simulink model "simulator_prototype"  (R2021b)
(part 12 of 12)

et761 = (t2307.*(-t6196+t6428+t3055.*(-t4494-t4495+t4799+t4823+t3976.*(t2694-t2701+t3036-t3043).*4.0e-8+t3980.*(t2694-t2701+t3036-t3043).*2.4e-7)))./2.0+(t7799.*(t1861-t3221))./2.0+(t3216.*(-t5828-t5829+t6593+t6596+t22.*t6699.*(t3242-t3554)+t28.*t6696.*(t3242-t3554)))./2.0;
et762 = (t3503.*(t6287+t4031.*(t4795+t4801+t4808+t3976.*(t2694-t2701+t3036-t3043).*5.7e-7)+t4026.*(-t4494-t4495+t4799+t4823+t3976.*(t2694-t2701+t3036-t3043).*4.0e-8+t3980.*(t2694-t2701+t3036-t3043).*2.4e-7)))./2.0;
et763 = (t3915.*(t6872+t6058.*(t1896-t3239)+t4019.*(t3435-t3448+t4615+t4619+t3976.*(t1896-t3239).*5.7e-7+t3980.*(t1896-t3239).*4.0e-8)))./2.0;
et764 = (t3217.*(t6251-t6997-t7310+t7388+t7554+t4880.*(t3435-t3448+t4615+t4619+t3976.*(t1896-t3239).*5.7e-7+t3980.*(t1896-t3239).*4.0e-8)))./2.0+t4215.*t5279.*(t2694-t2701+t3036-t3043).*5.43845e-3;
et765 = t3810.*t6011.*(t2694-t2701+t3036-t3043).*5.43845e-3+t3951.*t6647.*(t2694-t2701+t3036-t3043).*3.633675e-3+t3810.*t3934.*(et753+et754+et755+et756).*5.43845e-3+et757.*et758+t3934.*t5771.*(t1513+t1879+t2598+t2820+t2834+t3117+t3118).*3.633675e-3;
et766 = t50.*t189.*(t5618+t6429-t6902+t3055.*(t4795+t4801+t4808+t3976.*(t2694-t2701+t3036-t3043).*5.7e-7)+t6384.*(t1477-t2502)).*4.771516396025243e-17;
et767 = t5309+t5438+t6275+t6278+t7019+t7027+t7575+t7577-t7579+t7723+t7781+t7783+t7811-t7813-t7907+t7934-t7936+(t2994.*(-t6772+t6776+t3055.*(-t3434+t4606+t3980.*(t1896-t3239).*1.02e-6)))./2.0+(t7461.*(t1456-t2355))./2.0+(t7524.*(t11.*((t237.*(t42-t43))./9.007199254740992e+15+t15.*(-t1881+t3121+t3276))+t16.*(-t1901+t3122+t3277)))./2.0;
et768 = (t3047.*(t6462-t6464-t6766-t6767+t3055.*(t4809+t3976.*(t2694-t2701+t3036-t3043).*1.02e-6)+t5572.*(t1477-t2502)))./2.0;
et769 = t3704+t3707-t3863+t4904+t4912-t5154+t5155-t5186+t3370.*(t1477-t2502).*9.3e-7+t4031.*(t3512-t4006).*9.0e-8+t12.*t3980.*(t3242-t3554).*9.0e-8;
et770 = t17.*t3980.*(t3242-t3554).*9.3e-7;
et771 = t6736+t6778+t6779+t6783+t6787-t7024-t7025+t7205+t7207+t7398+(t3395.*(et769+et770))./2.0+(t5857.*(t4673+t2363.*(t3566.*1.838876e-2+t4109-t4110+t28.*(t1896-t3239).*9.99471e-3).*7.26735e-3))./2.0+(t5792.*(t1477-t2502))./2.0;
et772 = (t3055.*(t4876+t4905+t4906+t3055.*(t1456-t2355).*1.02e-6+t3047.*(t1477-t2502).*1.02e-6+t3976.*(t3242-t3554).*1.02e-6))./2.0;
et773 = t3704+t3707-t3863+t4904+t4912-t5154+t5155-t5186+t3370.*(t1477-t2502).*9.3e-7+t4031.*(t3512-t4006).*9.0e-8+t12.*t3980.*(t3242-t3554).*9.0e-8;
et774 = t17.*t3980.*(t3242-t3554).*9.3e-7;
et775 = t6738+t6778+t6779+t6783+t6787-t7024-t7025+t7205+t7207+t7398+(t3395.*(et773+et774))./2.0+(t5858.*(t4673+t2363.*(t3566.*1.838876e-2+t4109-t4110+t28.*(t1896-t3239).*9.99471e-3).*7.26735e-3))./2.0+(t5792.*(t1477-t2502))./2.0;
et776 = (t3055.*(t4876+t4905+t4906+t3055.*(t1456-t2355).*1.02e-6+t3047.*(t1477-t2502).*1.02e-6+t3976.*(t3242-t3554).*1.02e-6))./2.0;
et777 = t707+t708-t721-t722-t749+t762+t768-t777-t792-t793-t801-t802-t808+t813-t819+t821-t1629+t1637-t1640-t1641-t1659-t1661+t1666+t1667+t1683+t1692+t1705-t1712+t1758+t1759+t1775+t1776+t1973+t1993+t1994+t2023+t2053+t2060-t2089-t2090+t2098+t2099-t8.*t9.*t15.*t50.*t189.*3.670836568391568e-22;
et778 = t10.*t13.*t14.*t50.*t189.*(-3.279367663374749e-19)-t8.*t9.*t11.*t15.*t50.*t189.*7.075931802640439e-19;
et779 = t8.*t11.*t14.*t15.*t50.*t189.*(-1.190170786299927e-18)-t9.*t11.*t13.*t15.*t50.*t189.*1.190170786299927e-18;
et780 = t13.*t14.*t15.*t16.*t50.*t189.*(-3.226512155691387e-19);
et781 = -t5343-t5565-t5813-t5851+t5876-t5880+t6066+t6095+t6174+t6223-t6425+t6460-t6469+t6482+t6702+t6708-t6962-t6964+t6995+t7114-t7159-t7161+t7420;
et782 = (t5278.*(t350+t366-t1205+t1210-t1217-t1218-t2147+t2152+t2154+t2155-t3405-t3409-t3420-t3739+t3746+t26.*t50.*t202.*(t46-t47).*8.687615694748404e-39))./2.0;
et783 = (t3500.*(t4573.*(t2813-t2835+t12.*(t1456-t2355).*1.02e-6+t17.*(t1456-t2355).*9.0e-8)+t4577.*(-t2804+t2838+t3109+t17.*(t1456-t2355).*9.3e-7)+t3133.*(t3242-t3554)))./2.0+(t5026.*(et777+et778+et779+et780))./2.0+(t6916.*(t1861-t3221))./2.0;
et784 = (t6647.*(t3359-t3670+t22.*(t3242-t3554).*1.33637554986e-4+t28.*(t3242-t3554).*7.26350557185e-5))./2.0+(t3502.*(t3993+t4240-t4332+t4464+t4031.*(t2801-t2850)+t4026.*(t335-t1539-t2831+t2851)))./2.0;
et785 = (t5949.*(t4843+t5108+t2307.*(t642+t643-t667+t674+t1587+t1606+t1608+t1609+t2295+t2671+t2683+t2684-t2695+t3279+t3297-t3303+t3597+t3603+t3609-t3614+t4053+t4054)+t2297.*(t2292+t3290+t3524.*1.838876e-2-t3591+t3592+t3611+t16.*(t1861-t3221).*3.131399999999998e-4+t16.*t17.*(t1861-t3221).*9.99471e-3)))./2.0;
et786 = t1288+t1289+t1302+t1303-t1319-t1320+t1336-t1348+t1350+t1351-t1360+t1369-t1378+t1396-t1425+t1435-t2174+t2183-t2187+t2193-t2194-t2195+t2199-t2203-t2215+t2219-t2222-t2223+t2239+t2240-t2256-t2257+t2555+t2556+t2572+t2583-t2605-t2606+t2612+t2613-t2618-t2619+t2651+t2652;
et787 = t18.*t19.*t20.*t50.*t202.*(-3.566935413776081e-21);
et788 = t24.*t25.*t26.*t50.*t202.*(-3.992732227073824e-24);
et789 = t18.*t19.*t26.*t27.*t50.*t202.*(-3.509445006623964e-21);
et790 = t21.*t24.*t25.*t26.*t50.*t202.*(-7.696420262413979e-21);
et791 = -t5430+t5493-t5496+t6086-t6112+t6149+t6151./2.0+t6156-t6192+t6194-t6231+t6237+t6283+t6580+t6594+t6611+t6613-t6645-t6648-t6705-t6742+t6744-t7118-t7125+t7170+t7176-t7326+t7328+t7410+(t4950.*(et786+et787+et788+et789+et790))./2.0+(t7092.*(t1477-t2502))./2.0;
et792 = (t3055.*(t3131+t3132+t3171+t3446-t4281-t4282-t4301+t4303-t4308+t4310-t4583-t4594+t4623+t4639+t2388.*(t1456-t2355).*4.0e-8+(t3543.*(t1861-t3221))./1.0e+8+(t3500.*(t1896-t3239))./1.0e+8-t11.*t2297.*t2363.*2.4e-7))./2.0;
et793 = (t2363.*(t3157+t3158+t3386-t4299-t4300-t4562+t4567+t3543.*(t1861-t3221).*6.2e-7+t3500.*(t1896-t3239).*6.2e-7-(t11.*(t1861-t3221).*(t1896-t3239))./1.0e+8-(t11.*t2297.*t2363)./1.0e+8-(t11.*t3502.*t3547)./1.0e+8))./2.0+(t5859.*(t4927+t5198-t5762-t6392))./2.0;
et794 = (t21.*t2363.*(-t3434+t4606+t3980.*(t1896-t3239).*1.02e-6))./2.0;
et795 = t1288+t1289+t1302+t1303-t1319-t1320+t1336-t1348+t1350+t1351-t1360+t1369-t1378+t1396-t1425+t1435-t2174+t2183-t2187+t2193-t2194-t2195+t2199-t2203-t2215+t2219-t2222-t2223+t2239+t2240-t2256-t2257+t2555+t2556+t2572+t2583-t2605-t2606+t2612+t2613-t2618-t2619+t2651+t2652;
et796 = t18.*t19.*t20.*t50.*t202.*(-3.566935413776081e-21);
et797 = t24.*t25.*t26.*t50.*t202.*(-3.992732227073824e-24);
et798 = t18.*t19.*t26.*t27.*t50.*t202.*(-3.509445006623964e-21);
et799 = t21.*t24.*t25.*t26.*t50.*t202.*(-7.696420262413979e-21);
et800 = -t5430+t5493-t5496+t6086-t6112+t6149+t6151./2.0+t6156-t6192+t6194-t6233+t6239+t6283+t6580+t6594+t6611+t6613-t6646-t6649-t6705-t6742+t6744-t7118-t7125+t7170+t7176-t7326+t7328+t7412+(t4950.*(et795+et796+et797+et798+et799))./2.0+(t7092.*(t1477-t2502))./2.0;
et801 = (t3055.*(t3131+t3132+t3171+t3446-t4281-t4282-t4301+t4303-t4308+t4310-t4583-t4594+t4623+t4639+t2388.*(t1456-t2355).*4.0e-8+(t3543.*(t1861-t3221))./1.0e+8+(t3500.*(t1896-t3239))./1.0e+8-t11.*t2297.*t2363.*2.4e-7))./2.0;
et802 = (t2363.*(t3157+t3158+t3386-t4299-t4300-t4562+t4567+t3543.*(t1861-t3221).*6.2e-7+t3500.*(t1896-t3239).*6.2e-7-(t11.*(t1861-t3221).*(t1896-t3239))./1.0e+8-(t11.*t2297.*t2363)./1.0e+8-(t11.*t3502.*t3547)./1.0e+8))./2.0+(t5860.*(t4927+t5198-t5762-t6392))./2.0;
et803 = (t21.*t2363.*(-t3434+t4606+t3980.*(t1896-t3239).*1.02e-6))./2.0;
et804 = -t5344-t5568+t5679+t5689+t5925+t5927-t5966+t5976+t5980-t6241+t6295+t6367+t6528+t6540+t7028+t7031-t7040+t7300+t7302-t7363+t7612+t7616;
et805 = (t4118.*(t4573.*(t2813-t2835+t12.*(t1456-t2355).*1.02e-6+t17.*(t1456-t2355).*9.0e-8)+t4577.*(-t2804+t2838+t3109+t17.*(t1456-t2355).*9.3e-7)+t3133.*(t3242-t3554)))./2.0;
et806 = (t6651.*(t4814.*(t1861-t3221)+t2297.*(t642+t643-t667+t674+t1587+t1606+t1608+t1609+t2295+t2671+t2683+t2684-t2695+t3279+t3297-t3303+t3597+t3603+t3609-t3614+t4053+t4054)))./2.0+(t5809.*(t951+t10.*(-t1881+t3121+t3276)))./2.0+((t1861-t3221).*(t4658+t4719+t5240+t5262-t3483.*(t1005+t20.*(t1941-t3315+t39.*t1022.*(t855-t878).*2.196325630278387e-1))-t3431.*(t1896-t3239)))./2.0+(t3808.*t5645.*(t2674-t2676+t3022-t3027))./2.0;
et807 = (t3925.*t5946.*(t2674-t2676+t3022-t3027))./2.0;
et808 = -t5344-t5568+t5679+t5689+t5925+t5927-t5966+t5978+t5980-t6241+t6299+t6367+t6528+t6540+t7028+t7031-t7040+t7300+t7302-t7363+t7614+t7618;
et809 = (t4118.*(t4573.*(t2813-t2835+t12.*(t1456-t2355).*1.02e-6+t17.*(t1456-t2355).*9.0e-8)+t4577.*(-t2804+t2838+t3109+t17.*(t1456-t2355).*9.3e-7)+t3133.*(t3242-t3554)))./2.0;
et810 = (t6651.*(t4814.*(t1861-t3221)+t2297.*(t642+t643-t667+t674+t1587+t1606+t1608+t1609+t2295+t2671+t2683+t2684-t2695+t3279+t3297-t3303+t3597+t3603+t3609-t3614+t4053+t4054)))./2.0+(t5809.*(t951+t10.*(-t1881+t3121+t3276)))./2.0+((t1861-t3221).*(t4658+t4719+t5240+t5262-t3483.*(t1005+t20.*(t1941-t3315+t39.*t1022.*(t855-t878).*2.196325630278387e-1))-t3431.*(t1896-t3239)))./2.0+(t3808.*t5646.*(t2674-t2676+t3022-t3027))./2.0;
et811 = (t3925.*t5949.*(t2674-t2676+t3022-t3027))./2.0;
et812 = t5456+t5457+t7237+t7242+t7246+t7250+t7453+t7498+t7502+t7546+t7701+t7740+t7741-t7766+t7833+(t3047.*(t5490+t6190-t6193-t6609-t6610+t5405.*(t1477-t2502)))./2.0+(t3991.*(t5713+t5714-t6443-t6719-t6722+t6102.*(t3563-t4051)))./2.0+(t3980.*(t5691+t6884-t6886-t7353-t7354+t6065.*(t3242-t3554)))./2.0+(t7426.*(t1456-t2355))./2.0+(t3991.*(t6263-t6887+t6888-t7355+t7307.*(t3563-t4051)+t21.*t3547.*(-t3434+t4606+t3980.*(t1896-t3239).*1.02e-6)))./2.0;
et813 = (t11.*t7523.*(t1861-t3221))./2.0;
et814 = t31.*(et710+et711+et712+et713+et714+et715+et716+et717+et718+et719+et720+et721+et722+et723+et724+et725)+t29.*t7835+t30.*t7836+t32.*(et730+et731+et732+et733+et734+et735+et736+et737+et738+et739)-t33.*(et747+et748+et749+et750);
et815 = -t34.*(t7589+t7647+t7648+t7861+t7891+t7892-(t2297.*t7796)./2.0+(t3047.*t7714)./2.0-(t3502.*t7826)./2.0-(t3980.*t7755)./2.0-(t3991.*t7756)./2.0+((t1861-t3221).*(t7182-t7187+t4577.*(t3846-t5169-t5184+t5185+t3055.*(t2337+t12.*(t1456-t2355)).*9.3e-7+t4553.*(t3242-t3554).*9.3e-7)+t4573.*(t3840+t3862-t5164+t5167-t5183+t5189)))./2.0)+dq3.*dq4.*(et759+et760+et761+et762+et763+et764+et765+et766);
et816 = -dq3.*dq6.*(et767+et768)-dq1.*dq6.*(et771+et772)-dq2.*dq6.*(et775+et776)-dq5.*dq6.*(t5370-t5372-t7256+t7260+t7264+t7719+t7771+(t7755.*(t1861-t3221))./2.0+(t6711.*(t4675-t5454))./2.0).*2.0+dq3.*dq4.*(t4559+t4713+t5283+t5381+t5460+t5499+t5569+t5607+t5954+t5955+t6172+t6178+t6564+t6565+t6983+t6989+t7059+t7066+t7345+t7347+t7409+t7428+t7447+t7448+t7509+t7510+t7676+t7677+t7679+t7680+t7695+t7696+t7762+t7763+t7841+t7842+t7849+t7850+t7869+t7877+t7897+t7898+t7913+t7914)+dq1.*dq2.*t7963+dq1.*dq2.*t7964+dq1.*dq6.*t7961+dq2.*dq6.*t7962+dq1.*dq4.*t7977+dq1.*dq3.*t7985+dq2.*dq3.*t7986-dq2.*dq4.*(et781+et782+et783+et784+et785);
et817 = dq3.*dq6.*(t5296-t5439-t6305+t7080+t7084+t7586+t7650+t7651+t7775+t7888+t7890+t7944+t7955+t7956+(t7755.*(t2674-t2676+t3022-t3027))./2.0+((t4673+t2363.*(t3566.*1.838876e-2+t4109-t4110+t28.*(t1896-t3239).*9.99471e-3).*7.26735e-3).*(t2674-t2676+t3022-t3027).*(t1488+t1874+t2519+t2740+t2747+t3096+t3097))./2.0);
et818 = dq4.*dq5.*(t5433+t5434+t7442+t7454+t7487+t7489+t7501+t7507+t7514+t7516+t7542+t7545+t7830+t7832+t7839+t7840+t7846+t7847).*-2.0+dq4.*dq6.*(t5437+t5464+t7228+t7231+t7253+t7254+t7584+t7633+t7635+t7718+t7768+t7769+t7854+t7859+t7864+t7866+t7885+t7887)+dq3.*dq5.*(t5537+t5542+t7443+t7456+t7518+t7519+t7557+t7559+t7686+t7687+t7692+t7694+t7902+t7906+t7922+t7923+t7931+t7933).*2.0+dq1.*dq4.*(et791+et792+et793+et794)+dq2.*dq4.*(et800+et801+et802+et803)-dq1.*dq3.*(et804+et805+et806+et807)-dq2.*dq3.*(et808+et809+et810+et811)-dq4.*dq6.*(et812+et813);
et819 = t5548+t5550+t7219+t7220+t7221+t7222+t7699+t7732+t7734-(t3047.*(-t5453+t6371-t6616+t6617+t3395.*(t3428-t3432-t4570+t4576+t4582-t4603)+t3055.*(-t3080+t4100+t11.*t3236.*(t1861-t3221).*1.02e-6)))./2.0+(t3991.*(t5411-t5563+t6762-t6765+t4604.*(t3428-t3432-t4570+t4576+t4582-t4603)+t6244.*(t3563-t4051)))./2.0-(t3216.*t7862)./2.0-(t3217.*t7863)./2.0-(t3980.*t7748)./2.0;
et820 = t50.*t189.*(t5816-t6360-t7032+t7033+t7367-t7369).*4.771516396025243e-17+(t11.*t2297.*t7426)./2.0-(t11.*t3502.*t7470)./2.0-(t11.*t7469.*(t1861-t3221))./2.0;
et821 = -t2306-t2317+t3145+t3148+t35.*t941.*t948.*(t850-t874).*3.775747223193135e-1;
et822 = t36.*t941.*t948.*(t850-t874).*2.244797987218524e-1;
et823 = -t5393-t5395+t5758+t5759+t5760+t5761+t7787+t7788+(t2994.*t7461)./2.0+(t3047.*t7924)./2.0-(t3910.*t7951)./2.0+(t3980.*t7939)./2.0-(t3991.*t7940)./2.0-(t4838.*t7544)./2.0+(t4879.*t7630)./2.0-((t2674-t2676+t3022-t3027).*(t7211-t7238-t7240+t7662+t7663+t5792.*(t4165+t27.*(t1959-t3313+t38.*t1022.*(t855-t878).*2.196325630278387e-1))))./2.0;
et824 = (t7548.*(t11.*((t237.*(t42-t43))./9.007199254740992e+15+t15.*(-t1881+t3121+t3276))+t16.*(-t1901+t3122+t3277)))./2.0+(t7631.*(et821+et822))./2.0;
et825 = t5793+t5796+t4577.*(t4618+t4634-t12.*t2363.*t3047.*9.0e-8-t17.*t2363.*t3047.*9.3e-7+t12.*t3980.*(t1896-t3239).*9.0e-8+t17.*t3980.*(t1896-t3239).*9.3e-7);
et826 = t4573.*(t4617+t4635-t12.*t2363.*t3047.*1.02e-6-t17.*t2363.*t3047.*9.0e-8+t12.*t3980.*(t1896-t3239).*1.02e-6+t17.*t3980.*(t1896-t3239).*9.0e-8);
et827 = t22.*t6675.*(t3242-t3554)+t28.*t6674.*(t3242-t3554);
et828 = t3704+t3707-t3863+t4904+t4912-t5154+t5155-t5186+t3370.*(t1477-t2502).*9.3e-7+t4031.*(t3512-t4006).*9.0e-8+t12.*t3980.*(t3242-t3554).*9.0e-8;
et829 = t17.*t3980.*(t3242-t3554).*9.3e-7;
et830 = t1861-t3221;
et831 = -t5939-t6747+t4577.*(et828+et829)+t4573.*(t3703+t3708-t3856+t4903+t4911-t5153+t5161-t5190+t12.*t4887+t3370.*(t1477-t2502).*9.0e-8+t4031.*(t3512-t4006).*1.02e-6+t17.*t3980.*(t3242-t3554).*9.0e-8)+t22.*t6993.*(t3242-t3554)+t28.*t6992.*(t3242-t3554);
et832 = 1.0./2.0;
et833 = t5580+t5581+t6376-t6724-t6725;
et834 = t3395.*(t4618+t4634-t12.*t2363.*t3047.*9.0e-8-t17.*t2363.*t3047.*9.3e-7+t12.*t3980.*(t1896-t3239).*9.0e-8+t17.*t3980.*(t1896-t3239).*9.3e-7);
et835 = t5370-t5372-t7256+t7260+t7264+t7719+t7771-(t2297.*(t7022+t7023+t7394+t7397-t5792.*(t1477-t2502)-t3055.*(t4876+t4905+t4906+t3055.*(t1456-t2355).*1.02e-6+t3047.*(t1477-t2502).*1.02e-6+t3976.*(t3242-t3554).*1.02e-6)))./2.0-(t3502.*t7883)./2.0-(t3976.*t7523)./2.0;
et836 = t4001.*t7524.*(-1.0./2.0)-(t3991.*t7795)./2.0+(t7755.*(t1861-t3221))./2.0+(t6711.*(t4675-t5454))./2.0+(t3980.*(et825+et826+et827))./2.0+et830.*et831.*et832-((t1456-t2355).*(-t6772+t6776+t3055.*(-t3434+t4606+t3980.*(t1896-t3239).*1.02e-6)))./2.0-(t3047.*(et833+et834))./2.0;
et837 = t3704+t3707-t3863+t4904+t4912-t5154+t5155-t5186+t3370.*(t1477-t2502).*9.3e-7+t4031.*(t3512-t4006).*9.0e-8+t12.*t3980.*(t3242-t3554).*9.0e-8;
et838 = t17.*t3980.*(t3242-t3554).*9.3e-7;
et839 = t6736+t6778+t6779+t6783+t6787-t7024-t7025+t7205+t7207+t7398+(t3395.*(et837+et838))./2.0+(t5857.*(t4673+t2363.*(t3566.*1.838876e-2+t4109-t4110+t28.*(t1896-t3239).*9.99471e-3).*7.26735e-3))./2.0+(t5792.*(t1477-t2502))./2.0;
et840 = (t3055.*(t4876+t4905+t4906+t3055.*(t1456-t2355).*1.02e-6+t3047.*(t1477-t2502).*1.02e-6+t3976.*(t3242-t3554).*1.02e-6))./2.0;
et841 = t3704+t3707-t3863+t4904+t4912-t5154+t5155-t5186+t3370.*(t1477-t2502).*9.3e-7+t4031.*(t3512-t4006).*9.0e-8+t12.*t3980.*(t3242-t3554).*9.0e-8;
et842 = t17.*t3980.*(t3242-t3554).*9.3e-7;
et843 = t6738+t6778+t6779+t6783+t6787-t7024-t7025+t7205+t7207+t7398+(t3395.*(et841+et842))./2.0+(t5858.*(t4673+t2363.*(t3566.*1.838876e-2+t4109-t4110+t28.*(t1896-t3239).*9.99471e-3).*7.26735e-3))./2.0+(t5792.*(t1477-t2502))./2.0;
et844 = (t3055.*(t4876+t4905+t4906+t3055.*(t1456-t2355).*1.02e-6+t3047.*(t1477-t2502).*1.02e-6+t3976.*(t3242-t3554).*1.02e-6))./2.0;
et845 = t5296-t5439-t6305+t7080+t7084-t7579+t7775+t7888+t7890-t7907+t7934-t7936+(t2994.*(-t6772+t6776+t3055.*(-t3434+t4606+t3980.*(t1896-t3239).*1.02e-6)))./2.0+(t7524.*(t11.*((t237.*(t42-t43))./9.007199254740992e+15+t15.*(-t1881+t3121+t3276))+t16.*(-t1901+t3122+t3277)))./2.0+(t7755.*(t2674-t2676+t3022-t3027))./2.0;
et846 = ((t4673+t2363.*(t3566.*1.838876e-2+t4109-t4110+t28.*(t1896-t3239).*9.99471e-3).*7.26735e-3).*(t2674-t2676+t3022-t3027).*(t1488+t1874+t2519+t2740+t2747+t3096+t3097))./2.0;
et847 = t34.*((t3047.*t7796)./2.0-(t3991.*t7826)./2.0+(t3980.*(t7182-t7187+t4577.*(t3846-t5169-t5184+t5185+t3055.*(t2337+t12.*(t1456-t2355)).*9.3e-7+t4553.*(t3242-t3554).*9.3e-7)+t4573.*(t3840+t3862-t5164+t5167-t5183+t5189)))./2.0)+t29.*t7710+t30.*t7713-t32.*(et819+et820)+t31.*(et823+et824)+t33.*(et835+et836);
et848 = -dq3.*dq4.*(t5404+t5544+t6228+t6230+t6971+t6975+t7466+t7564+t7568+t7583+t7645+t7646+t7721+t7765+t7778+t7780+t7821+t7822+t7943+t7953+t7954)+dq4.*dq6.*(-t7585+t7636+t7855+t7873+t7874+(t11.*t7630.*(t1861-t3221))./2.0).*2.0+dq5.*dq6.*(t7589+t7647+t7648+t7861+t7891+t7892).*2.0+dq3.*dq6.*(t7587-t7660+t7945+t7957-t7958+(t7631.*(t11.*((t237.*(t42-t43))./9.007199254740992e+15+t15.*(-t1881+t3121+t3276))+t16.*(-t1901+t3122+t3277)))./2.0).*2.0+dq1.*dq5.*(et839+et840)+dq2.*dq5.*(et843+et844);
et849 = -dq1.*dq4.*(t5819+t6362-t6635+t6639+t6640+t6643-t6692-t6694+t7037+t7038+t7156+t7370+t7373+(t6682.*(-t4045+t4049+t12.*(t1861-t3221).*1.838876e-2+t17.*(t1861-t3221).*9.99471e-3))./2.0);
et850 = -dq2.*dq4.*(t5819+t6362-t6635+t6639+t6640+t6643-t6693-t6695+t7037+t7038+t7156+t7370+t7373+(t6682.*(-t4045+t4049+t12.*(t1861-t3221).*1.838876e-2+t17.*(t1861-t3221).*9.99471e-3))./2.0)+dq1.*dq2.*t7711+dq1.*dq2.*t7712+dq1.*dq3.*t7948+dq2.*dq3.*t7949+dq1.*dq4.*t7959+dq2.*dq4.*t7960-dq1.*dq5.*t7961-dq2.*dq5.*t7962+dq1.*dq3.*t7971+dq2.*dq3.*t7972;
et851 = dq4.*dq5.*(t5456+t5457+t7237+t7242+t7246+t7250+t7498+t7502+t7584+t7633+t7635+t7701+t7740+t7741-t7766+t7854+t7864+t7866+(t3047.*(t5490+t6190-t6193-t6609-t6610+t5405.*(t1477-t2502)))./2.0+(t3991.*(t5713+t5714-t6443-t6719-t6722+t6102.*(t3563-t4051)))./2.0+(t7426.*(t1456-t2355))./2.0)-dq3.*dq4.*(t5399+t5545+t6250+t6261+t7000+t7001+t7430+t7529+t7530+t7744+t7745+t7870+t7872+t7879+t7917+t7918);
et852 = -dq4.*dq5.*(t5437+t5464+t7228+t7231+t7253+t7254+t7453+t7546+t7718+t7768+t7769+t7833+t7859+t7885+t7887+(t3980.*(t5691+t6884-t6886-t7353-t7354+t6065.*(t3242-t3554)))./2.0+(t3991.*(t6263-t6887+t6888-t7355+t7307.*(t3563-t4051)+t21.*t3547.*(-t3434+t4606+t3980.*(t1896-t3239).*1.02e-6)))./2.0+(t11.*t7523.*(t1861-t3221))./2.0);
et853 = dq3.*dq5.*(t5309+t5438+t6275+t6278+t7019+t7027+t7575+t7577+t7586+t7650+t7651+t7723+t7781+t7783+t7811-t7813+t7944+t7955+t7956+(t7461.*(t1456-t2355))./2.0+(t3047.*(t6462-t6464-t6766-t6767+t3055.*(t4809+t3976.*(t2694-t2701+t3036-t3043).*1.02e-6)+t5572.*(t1477-t2502)))./2.0)-dq3.*dq5.*(et845+et846);
tau_c = real([et359+et360+et361+et362+et363+et364+et365+et366+et367+et368+et369;et430+et431+et432+et433+et434+et435+et436;et551+et552;et691+et692+et693+et694+et695+et696;et814+et815+et816+et817+et818;et847+et848+et849+et850+et851+et852+et853]);
end
